simulink model "X31dynamics_03"  (R2014b)
settings: Solver=ode45  StartTime=0.0  StopTime=20  RelTol=1e-3
InitFcn:
  | X31dynamics_03_init
undefined symbols (not defined in the file or in its folder): Newton, Raphson, X31_initC, X31_initR, X31_initX, X31_physical
libraries: QuaternionLib x9, cstblocks x7, simulink x2
settings Model: Creator=EwingKang  LastModifiedBy=5909
settings SolverCC: ZeroCrossAlgorithm=Adaptive
settings DataIOCC: SaveOutput=off  SaveTime=off
settings OptimizationCC: InlineParams=on
settings DebuggingCC: UnderspecifiedInitializationDetection=Classic  MergeDetectMultiDrivingBlocksExec=none  StateNameClashWarn=warning  StrictBusMsg=ErrorOnBusTreatedAsVector
settings ModelReferenceCC: ModelReferenceNumInstancesAllowed=Single  ModelReferencePassRootInputsByReference=off
settings SimscapeCC: EditingMode=Restricted

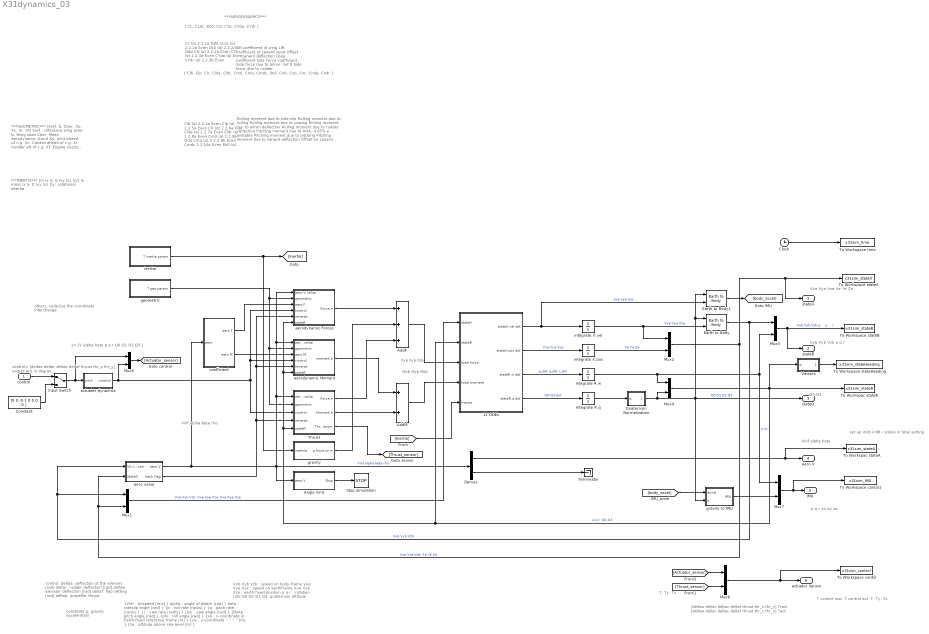
== system X31dynamics_03 ==
  note: Q0-Q3
  note: set up initX initR i sdone in total setting
  note: others:
      | code-lize the coordinate interchange
  note: constants
      | g: gravity acceleration
  note: control:
      |   deltaa: deflection of the ailerons [rad]
      |   deltar: rudder deflection [rad]
      |   deltae: elevator deflection [rad]
      |   deltaf: flap setting [rad]
      |   deltap: propeller thrust
  note: Vxb  Vyb Vzb : speed on body frame
      | Vxe Vye Vze  : speed on earthframe
      | Xxe Xye Xze  : earth fixed position
      | p q r               : rotation rate
      | Q0 Q1 Q2 Q3: quaternion attitude
  note: Vxb Vyb Vzb
      | p     q     r
  note: Vxe Vye Vze
      | Xe   Ye   Ze
  note: {Vinf    : airspeed [m/s]                                                  }
      |  alpha : angle of attack [rad]                                          }
      |  beta   : sideslip angle [rad]                                           }
      | {p    : roll rate [rad/s]                                                      }
      | {q    : pitch rate [rad/s]                                                   }
      | {r     : yaw rate [rad/s]                                                    }
      | {psi    : yaw angle [rad]                                                  }
      | {theta : pitch angle [rad]                                                }
      | {phi    : roll angle [rad]                                                   }
      | {xe   : x-coordinate in Earth-fixed reference frame [m]  }
      | {ye   : y-coordinate ''     ''          ''      ''  [m]                     }
      | {ze   : altitude above sea-level [m]                                }
  note: control= [deltaa deltar deltac deltaf thrust thr_z thr_y]
      | angles are in degree
  note: x= [V alpha beta p q r Q0 Q1 Q2 Q3 ]
  note: Mxb Myb Mzb
  note: Fxb Fyb Fzb
  note: Vinf
      | alpha
      | beta
      | rho
  note: ***AERODYNAMICS***
  note: ***INERTIA***
      | [m Ix Iy Iz Ixy Ixz Iyz]
      | m : mass
      | Ix Iy Iz Ixy Ixz Izy: rotational intertia
  note: ***GEOMETRIC***
      |  [Sref, b, Cbar, Xp, Xc, Xr, Xt]
      |
      | Sref : reference wing area
      | b: Wing span
      | Cbar: Mean aerodynamic chord
      | Xp: pilot ahead of c.g.
      | Xc: Canard ahead of c.g.
      | Xr: Rudder aft of c.g.
      | Xt: Engine nozzle after of c.g.
  note: Rolling moment due to side-slip
      | Rolling moment due to rolling
      | Rolling moment due to yawing
      | Rolling moment due to ailron deflection
      | Rolling moment due to rudder deflection
      |
      | Pitching moment due to AOA, 4.65% e unstable
      | Pitching moment due to pitching
      | Pitching moment due to canard deflection
      | Offset on canard deflection
      |
      | Yawing moment due to side-slip
      | Yawing moment due to rolling
      | Yawing moment due to yawing
      | Yawing moment due to ailron deflection
      | Yawing moment due to rudder deflection
  note: Lift coefficient of wing
      | Lift coefficient of canard input
      | Offset on canard deflection
      | Drag coefficient
      | Side Force coefficient
      | Side force due to ailron, set 0
      | Side force due to rudder
  note: Clb    (α) 2.2.4a Even
      | Clp    (α) 2.2.5a Even
      | Clr     (α) 2.2.6a Odd
      | Clda  (α) 2.2.7a Even
      | Cldr   (α) 2.2.8a Even
      |
      | Cm0  (α) 2.2.9a Odd
      | Cmq  (α) 3 2.2.9b Even
      | Cmdc      2.2.10a Even
      | Dc0   (α) 2.2.2/10b Odd
      |
      | Cnb  (α) 2.2.4b Even
      | Cnp  (α) 2.2.5b Odd
      | Cnr   (α) 2.2.6b Even
      | Cnda(α) 2.2.7b Even
      | Cndr (α) 2.2.8b Even
  note: CL     (α) 2.2.1a Odd
      | CLdc (α)  2.2.2a Even
      | Dc0   (α)  2.2.2/l0b Odd
      | CD     (α)  2.2.1b Even
      | CYb   (α) 2.2.3a Even
      | CYda (α)            Even
      | CYdr  (α) 2.2.3b Even
  note: [ CL, CLdc, Dc0, CD, CYp, CYda, CYdr ]
  note: [ Clb, Clp, Clr, Clda, Cldr, Cm0, Cmq, Cmdc, Dc0, Cnb, Cnp, Cnr, Cnda, Cndr ]
  note: Vinf
      | alpha
      | beta
  note: T, Ty, Tz
  note: [deltaa deltar deltac deltaf thrust thr_z thr_y] 7raw
      | [deltaa deltar deltac deltaf thrust thr_z thr_y] 7act
  note: 7 contorl raw, 7 control act, T, Ty, Tz
  note: p q r ax ay az
  control : Inport  PortDimensions=7
  12 ODEs : Subsystem
  AddF : Sum  Inputs=+++
  AddM : Sum
  Angle limit : Subsystem
  Clock : Clock
  Constant : Constant  Value=[0 0 -0.1 0 0 0 0 ]
  Demux : Demux  Outputs=[3 1 ]
  Earth to Body : QuaternionLib/Earth to Body
  Earth to Body1 : QuaternionLib/Earth to Body
  Input Switch : ManualSwitch
  Integrate R.q : Integrator  InitialCondition=X31_initR.q
  Integrate R.w : Integrator  InitialCondition=X31_initR.w
  Mux{1..7} (7 alike) : Mux  Inputs=2
  Quaternion Normalization : Subsystem
  Stop Simulation : Stop
  Terminator : Terminator
  Thrust : Subsystem
  To Workspac stateA : ToWorkspace  VariableName=x31sim_stateA  SaveFormat=Timeseries  SampleTime=-1
  To Workspac stateR : ToWorkspace  VariableName=x31sim_stateR  SaveFormat=Timeseries  SampleTime=-1
  To Workspace contol : ToWorkspace  VariableName=x31sim_control  SaveFormat=Timeseries  SampleTime=-1
  To Workspace contol1 : ToWorkspace  VariableName=x31sim_IMU  SaveFormat=Timeseries  SampleTime=-1
  To Workspace stateB : ToWorkspace  VariableName=x31sim_stateB  SaveFormat=Timeseries  SampleTime=-1
  To Workspace stateHeading : ToWorkspace  VariableName=x31sim_stateHeading  SaveFormat=Timeseries  SampleTime=-1
  To Workspace stateX : ToWorkspace  VariableName=x31sim_stateX  SaveFormat=Timeseries  SampleTime=-1
  To Workspace time : ToWorkspace  VariableName=x31sim_time  SaveFormat=Timeseries  SampleTime=-1
  Vectors : Subsystem
  actuater dynamics : Subsystem
  aero value : Subsystem
  aerodynamic Forces : Subsystem
  aerodynamic Moment : Subsystem
  coefficient : Subsystem
  geometric : Subsystem
  gravity : Subsystem
  gravity to IMU : Subsystem
  inertia : Subsystem
  integrate X.pos : Integrator  InitialCondition=X31_initX.pos
  integrate X.vel : Integrator  InitialCondition=X31_initX.vel
  stateX : Outport
  stateB : Outport  Port=2
  stateQ : Outport  Port=3
  aero V : Outport  Port=4
  IMU : Outport  Port=5
  actuator Sensor : Outport  Port=6
  wires:
  12 ODEs/1(stateX.vel dot) -> Earth to Body1/2, integrate X.vel/1  "axe aye aze"
  12 ODEs/3("stateR.w dot ") -> Integrate R.w/1  "p_dot q_dot r_dot"
  Mux2/1 -> To Workspace stateX/1, stateX/1, aero value/2(StateX), Mux1/2  "Vxe Vye Vze  Xe Ye Ze"
  Earth to Body/1 -> Mux3/1, aero value/1(Vb vector), Mux1/1  "Vxb Vyb Vzb"
  Mux1/1 -> 12 ODEs/1(stateX)  "Vxb Vyb Vzb  Vxe Vye Vze  Xxe Xye Xze"
  aerodynamic Forces/1(Force e) -> AddF/1
  gravity/1(g force on e) -> AddF/2
  aerodynamic Moment/1(moment b) -> AddM/1
  AddM/1 -> 12 ODEs/4(total moment)
  AddF/1 -> 12 ODEs/3(total force)
  geometric/1(7 geo param) -> Thrust/2(geometric), aerodynamic Moment/2(geometric), aerodynamic Forces/2(geometric)
  coefficient/1(aero F) -> aerodynamic Forces/3(aero F)
  Input Switch/1 -> actuater dynamics/1(cmd), Mux5/1
  aero value/1(aero V) -> coefficient/1(aero), aerodynamic Moment/1(aero V value), aerodynamic Forces/1(aero V value), Thrust/1(aero V value), Angle limit/1(aero V), Demux/1  "Vinf alpha beta rho"
  inertia/1(7 inertia param) -> [Inertia], gravity/1(inertria)
  Clock/1 -> To Workspace time/1
  aero value/2(back flag) -> aerodynamic Moment/5(reverse), aerodynamic Forces/5(reverse), Thrust/4(reverse)
  Mux4/1 -> To Workspac stateR/1, aerodynamic Moment/6(stateR), aerodynamic Forces/6(stateR), Thrust/5(stateR), 12 ODEs/2(stateR), Vectors/1(q)  "p q r  Q0-Q3"
  Quaternion Normalization/1(qnorm) -> Earth to Body1/1, Earth to Body/1, gravity to IMU/2(q), stateQ/1, Mux4/2  "Q0 Q1 Q2 Q3"
  integrate X.vel/1 -> Earth to Body/2, Mux2/1  "Vxe Vye Vze"
  Integrate R.w/1 -> Mux3/2, Mux7/1, Mux4/1  "p q r"
  Integrate R.q/1 -> Quaternion Normalization/1(q)
  actuater dynamics/1(control) -> aerodynamic Moment/4(control), aerodynamic Forces/4(control), Thrust/3(control), Mux5/2
  Mux5/1 -> [Actuator_sensor]
  [Inertia] -> 12 ODEs/5(Inertia)
  Mux3/1 -> To Workspace stateB/1, stateB/1  "Vxb Vyb Vzb p     q     r"
  Constant/1 -> Input Switch/2
  control/1 -> Input Switch/1
  coefficient/2(aero M) -> aerodynamic Moment/3(aero M)
  Thrust/2(Moment b) -> AddM/2
  Thrust/1(Force e) -> AddF/3
  Angle limit/1(Stop) -> Stop Simulation/1
  12 ODEs/2(stateX.pos dot) -> integrate X.pos/1  "Vxe Vye Vze"
  12 ODEs/4(stateR.q dot) -> Integrate R.q/1  "Q0-Q3 dot"
  integrate X.pos/1 -> Mux2/2  "Xe Ye Ze"
  Vectors/1(Vector) -> To Workspace stateHeading/1
  Demux/1 -> To Workspac stateA/1, aero V/1
  Demux/2 -> Terminator/1
  [Thrust_sensor] -> Mux6/2
  Thrust/3(Thrust sensor) -> [Thrust_sensor]
  [Actuator_sensor] -> Mux6/1
  Mux6/1 -> actuator Sensor/1, To Workspace contol/1
  Mux7/1 -> IMU/1, To Workspace contol1/1
  Earth to Body1/1 -> [body_accel]
  [body_accel] -> gravity to IMU/1(accel)
  gravity to IMU/1(IMU) -> Mux7/2

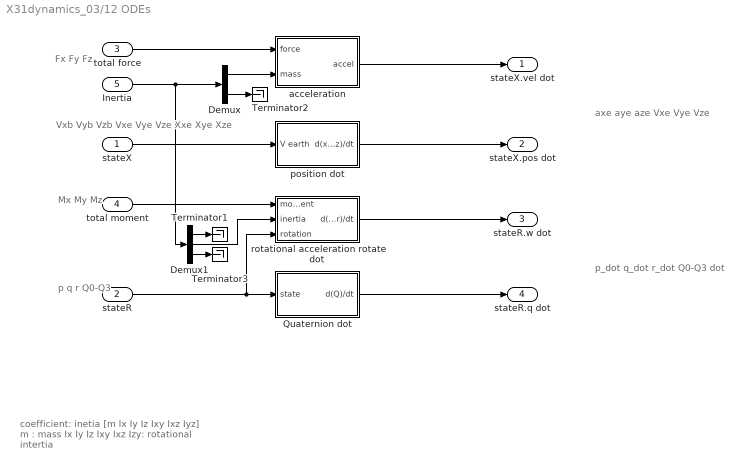
== system X31dynamics_03/12 ODEs ==
  note: p_dot q_dot r_dot
      | Q0-Q3 dot
  note: axe aye aze
      | Vxe Vye Vze
  note: Vxb Vyb Vzb Vxe Vye Vze Xxe Xye Xze
  note: Mx My Mz
  note: Fx Fy Fz
  note: p q r Q0-Q3
  note: coefficient: inetia
      | [m Ix Iy Iz Ixy Ixz Iyz]
      | m : mass
      | Ix Iy Iz Ixy Ixz Izy: rotational intertia
  stateX : Inport
  stateR : Inport  Port=2
  total force : Inport  Port=3
  total moment : Inport  Port=4
  Inertia : Inport  Port=5
  Demux : Demux  Outputs=[1 6]
  Demux1 : Demux  Outputs=[1 3 3]
  Quaternion dot : Subsystem
  Terminator1 : Terminator
  Terminator2 : Terminator
  Terminator3 : Terminator
  acceleration : Subsystem
  position dot : Subsystem
  rotational acceleration rotate dot : Subsystem
  stateX.vel dot : Outport
  stateX.pos dot : Outport  Port=2
  "stateR.w dot " : Outport  Port=3
  stateR.q dot : Outport  Port=4
  wires:
  Inertia/1 -> Demux1/1, Demux/1
  total moment/1 -> rotational acceleration rotate dot/1(moment)
  total force/1 -> acceleration/1(force)
  stateR/1 -> rotational acceleration rotate dot/3(rotation), Quaternion dot/1(state)
  acceleration/1(accel) -> stateX.vel dot/1
  position dot/1(d(xyz)/dt) -> stateX.pos dot/1
  rotational acceleration rotate dot/1(d(pqr)/dt) -> "stateR.w dot "/1
  stateX/1 -> position dot/1(V earth)
  Demux/1 -> acceleration/2(mass)
  Demux/2 -> Terminator2/1
  Demux1/2 -> rotational acceleration rotate dot/2(inertia)
  Demux1/1 -> Terminator1/1
  Demux1/3 -> Terminator3/1
  Quaternion dot/1(d(Q)/dt) -> stateR.q dot/1

== system X31dynamics_03/Angle limit ==
  note: Vinf
      | alpha
      | beta
      | rho
  aero V : Inport
  85 degree : simulink/Logic and Bit Operations/Compare To Constant  relop=>  const=85 * pi / 180  OutDataTypeStr=boolean
  85 degree1 : simulink/Logic and Bit Operations/Compare To Constant  relop=>  const=80 * pi / 180  OutDataTypeStr=boolean
  Abs : Abs
  Abs1 : Abs
  Any violation : Logic  Operator=OR  AllPortsSameDT=off  OutDataTypeStr=boolean
  Assertion : Assertion  AssertionFailFcn=warning('large angle in x31dynamics_03')  StopWhenAssertionFail=off
  Logical Operator : Logic  Operator=NOT  AllPortsSameDT=off  OutDataTypeStr=boolean
  alpha : Fcn  Expr=u(2)
  beta : Fcn  Expr=u(3)
  Stop : Outport
  wires:
  aero V/1 -> alpha/1, beta/1
  85 degree/1 -> Any violation/1
  alpha/1 -> Abs/1
  beta/1 -> Abs1/1
  85 degree1/1 -> Any violation/2
  Abs/1 -> 85 degree/1
  Abs1/1 -> 85 degree1/1
  Any violation/1 -> Logical Operator/1, Stop/1
  Logical Operator/1 -> Assertion/1

== system X31dynamics_03/Quaternion Normalization ==
  q : Inport  PortDimensions=4
  Product : Product  Inputs=*/  SaturateOnIntegerOverflow=on  RndMeth=Zero  InputSameDT=on  OutDataTypeStr=Inherit: Same as first input
  Square : Math  Operator=square  SaturateOnIntegerOverflow=on
  Square Root : Sqrt  Operator=signedSqrt  AlgorithmType=Newton-Raphson  SaturateOnIntegerOverflow=on
  Sum : Sum  Inputs=1  SaturateOnIntegerOverflow=on  InputSameDT=on  OutDataTypeStr=Inherit: Same as first input
  qnorm : Outport
  wires:
  Product/1 -> qnorm/1
  Square Root/1 -> Product/2
  Square/1 -> Sum/1
  Sum/1 -> Square Root/1
  q/1 -> Product/1, Square/1

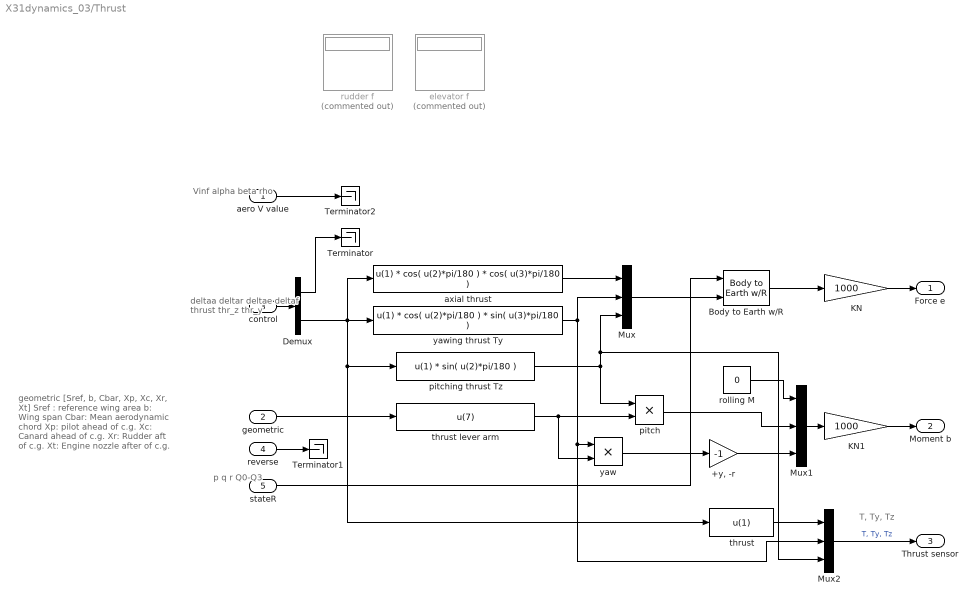
== system X31dynamics_03/Thrust ==
  note: T, Ty, Tz
  note: Vinf alpha beta rho
  note: p q r
      | Q0-Q3
  note: geometric
      |  [Sref, b, Cbar, Xp, Xc, Xr, Xt]
      |
      | Sref : reference wing area
      | b: Wing span
      | Cbar: Mean aerodynamic chord
      | Xp: pilot ahead of c.g.
      | Xc: Canard ahead of c.g.
      | Xr: Rudder aft of c.g.
      | Xt: Engine nozzle after of c.g.
  note: deltaa deltar deltae deltaf
      | thrust thr_z thr_y
  aero V value : Inport
  geometric : Inport  Port=2
  control : Inport  Port=3
  reverse : Inport  Port=4
  stateR : Inport  Port=5
  " thrust" : Fcn  Expr=u(1)
  "+y, -r" : Gain  Gain=-1
  Body to Earth w/R : QuaternionLib/Body to Earth w//R
  Demux : Demux  Outputs=[4 3]
  KN : Gain  Gain=1000
  KN1 : Gain  Gain=1000
  Mux : Mux  Inputs=3
  Mux1 : Mux  Inputs=3
  Mux2 : Mux  Inputs=3
  Terminator : Terminator
  Terminator1 : Terminator
  Terminator2 : Terminator
  axial thrust : Fcn  Expr="u(1) * cos( u(2)*pi/180  ) * cos( u(3)*pi/180  )"
  elevator f : Display  Commented=on
  pitch : Product
  pitching thrust Tz : Fcn  Expr=u(1) * sin( u(2)*pi/180 )
  rolling M : Constant  Value=0
  rudder f : Display  Commented=on
  thrust lever arm : Fcn  Expr=u(7)
  yaw : Product
  yawing thrust Ty : Fcn  Expr=u(1) * cos( u(2)*pi/180 ) * sin( u(3)*pi/180 )
  Force e : Outport
  Moment b : Outport  Port=2
  Thrust sensor : Outport  Port=3
  wires:
  control/1 -> Demux/1
  Body to Earth w/R/1 -> KN/1
  Demux/1 -> Terminator/1
  yawing thrust Ty/1 -> Mux/2, Mux2/2, yaw/1
  axial thrust/1 -> Mux/1
  pitching thrust Tz/1 -> Mux2/3, Mux/3, pitch/1
  Mux/1 -> Body to Earth w/R/2
  stateR/1 -> Body to Earth w/R/1
  Demux/2 -> " thrust"/1, pitching thrust Tz/1, axial thrust/1, yawing thrust Ty/1
  reverse/1 -> Terminator1/1
  aero V value/1 -> Terminator2/1
  geometric/1 -> thrust lever arm/1
  thrust lever arm/1 -> yaw/2, pitch/2
  yaw/1 -> "+y, -r"/1
  pitch/1 -> Mux1/2
  rolling M/1 -> Mux1/1
  Mux1/1 -> KN1/1
  KN/1 -> Force e/1
  KN1/1 -> Moment b/1
  "+y, -r"/1 -> Mux1/3
  Mux2/1 -> Thrust sensor/1  "T, Ty, Tz"
  " thrust"/1 -> Mux2/1

== system X31dynamics_03/Vectors ==
  q : Inport
  1,0,0 : Subsystem
  1,0,1 : Subsystem
  Body to Earth w/R1 : QuaternionLib/Body to Earth w//R
  Body to Earth w/R2 : QuaternionLib/Body to Earth w//R
  Mux6 : Mux  Inputs=2
  Vector : Outport
  wires:
  1,0,0/1(1,0,0) -> Body to Earth w/R1/2
  Body to Earth w/R1/1 -> Mux6/1
  q/1 -> Body to Earth w/R1/1, Body to Earth w/R2/1  "p q r  Q0-Q3"
  Mux6/1 -> Vector/1
  Body to Earth w/R2/1 -> Mux6/2
  1,0,1/1(0,1,0) -> Body to Earth w/R2/2

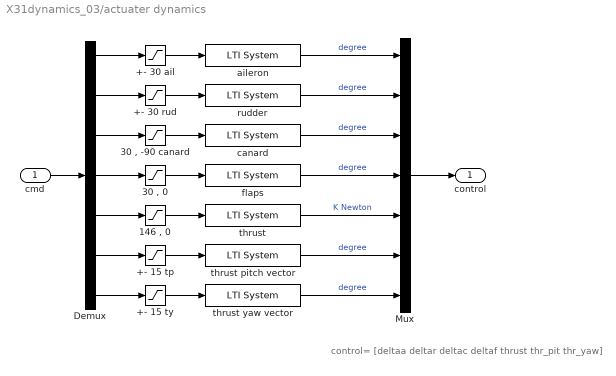
== system X31dynamics_03/actuater dynamics ==
  note: control= [deltaa deltar deltac deltaf thrust thr_pit thr_yaw]
  cmd : Inport
  +- 15 tp : Saturate  UpperLimit=15  LowerLimit=-15
  +- 15 ty : Saturate  UpperLimit=15  LowerLimit=-15
  +- 30 ail : Saturate  UpperLimit=30  LowerLimit=-30
  +- 30 rud : Saturate  UpperLimit=30  LowerLimit=-30
  "146 , 0" : Saturate  UpperLimit=146  LowerLimit=0
  "30 , -90 canard" : Saturate  UpperLimit=30  LowerLimit=-90
  "30 , 0" : Saturate  UpperLimit=30  LowerLimit=0
  Demux : Demux  Outputs=7
  Mux : Mux  Inputs=7
  aileron : cstblocks/LTI System  sys=tf(30,[1 30])  IC=[]
  canard : cstblocks/LTI System  sys=tf(30,[1 30])  IC=[]
  flaps : cstblocks/LTI System  sys=tf(30,[1 30])  IC=[]
  rudder : cstblocks/LTI System  sys=tf(30,[1 30])  IC=[]
  thrust : cstblocks/LTI System  sys=ss(-1/3, 1, 1/3, 0)  IC=[X31_initC.thrust*3]
  thrust pitch vector : cstblocks/LTI System  sys=tf(30,[1 30])  IC=[]
  thrust yaw vector : cstblocks/LTI System  sys=tf(30,[1 30])  IC=[]
  control : Outport
  wires:
  cmd/1 -> Demux/1
  Demux/4 -> "30 , 0"/1
  Demux/3 -> "30 , -90 canard"/1
  Demux/2 -> +- 30 rud/1
  Demux/1 -> +- 30 ail/1
  Demux/5 -> "146 , 0"/1
  Demux/6 -> +- 15 tp/1
  Demux/7 -> +- 15 ty/1
  thrust yaw vector/1 -> Mux/7  "degree"
  thrust pitch vector/1 -> Mux/6  "degree"
  thrust/1 -> Mux/5  "K Newton"
  flaps/1 -> Mux/4  "degree"
  canard/1 -> Mux/3  "degree"
  rudder/1 -> Mux/2  "degree"
  aileron/1 -> Mux/1  "degree"
  Mux/1 -> control/1
  +- 30 ail/1 -> aileron/1
  +- 30 rud/1 -> rudder/1
  "30 , -90 canard"/1 -> canard/1
  "30 , 0"/1 -> flaps/1
  "146 , 0"/1 -> thrust/1
  +- 15 tp/1 -> thrust pitch vector/1
  +- 15 ty/1 -> thrust yaw vector/1

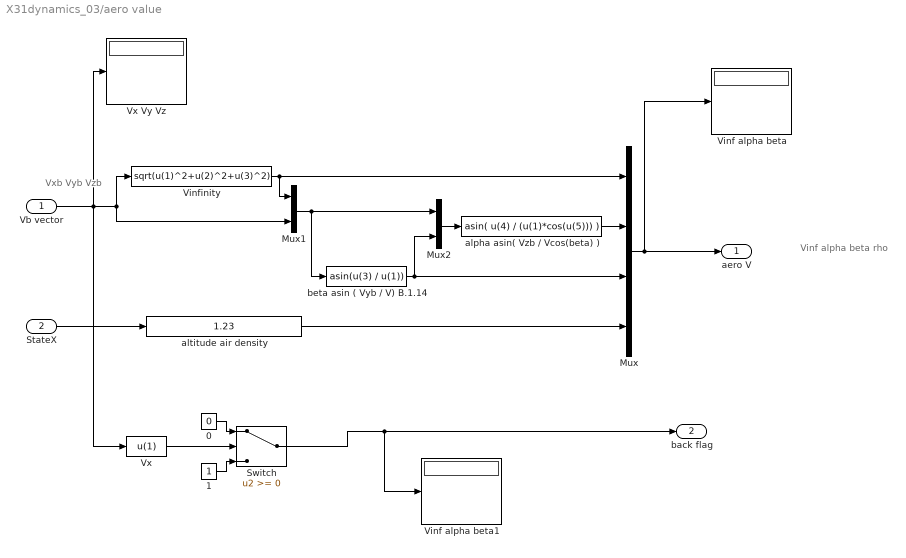
== system X31dynamics_03/aero value ==
  note: Vinf
      | alpha
      | beta
      | rho
  note: Vxb Vyb Vzb
  Vb vector : Inport
  StateX : Inport  Port=2
  0 : Constant  Value=0
  1 : Constant
  Mux : Mux
  Mux1 : Mux  Inputs=2
  Mux2 : Mux  Inputs=2
  Switch : Switch  ZeroCross=off
  Vinf alpha beta : Display
  Vinf alpha beta1 : Display
  Vinfinity : Fcn  Expr=sqrt(u(1)^2+u(2)^2+u(3)^2)
  Vx : Fcn  Expr=u(1)
  Vx Vy Vz : Display
  alpha asin( Vzb / Vcos(beta) ) : Fcn  Expr=asin( u(4) / (u(1)*cos(u(5))) )
  altitude air density : Fcn  Expr=1.23
  beta asin ( Vyb / V) B.1.14 : Fcn  Expr=asin(u(3) / u(1))
  aero V : Outport
  back flag : Outport  Port=2
  wires:
  Vb vector/1 -> Vx/1, Vx Vy Vz/1, Vinfinity/1, Mux1/2
  Vinfinity/1 -> Mux1/1, Mux/1
  beta asin ( Vyb / V) B.1.14/1 -> Mux/3, Mux2/2
  Mux/1 -> aero V/1, Vinf alpha beta/1
  alpha asin( Vzb / Vcos(beta) )/1 -> Mux/2
  Vx/1 -> Switch/2
  0/1 -> Switch/1
  1/1 -> Switch/3
  Switch/1 -> Vinf alpha beta1/1, back flag/1
  Mux1/1 -> beta asin ( Vyb / V) B.1.14/1, Mux2/1
  altitude air density/1 -> Mux/4
  StateX/1 -> altitude air density/1
  Mux2/1 -> alpha asin( Vzb / Vcos(beta) )/1

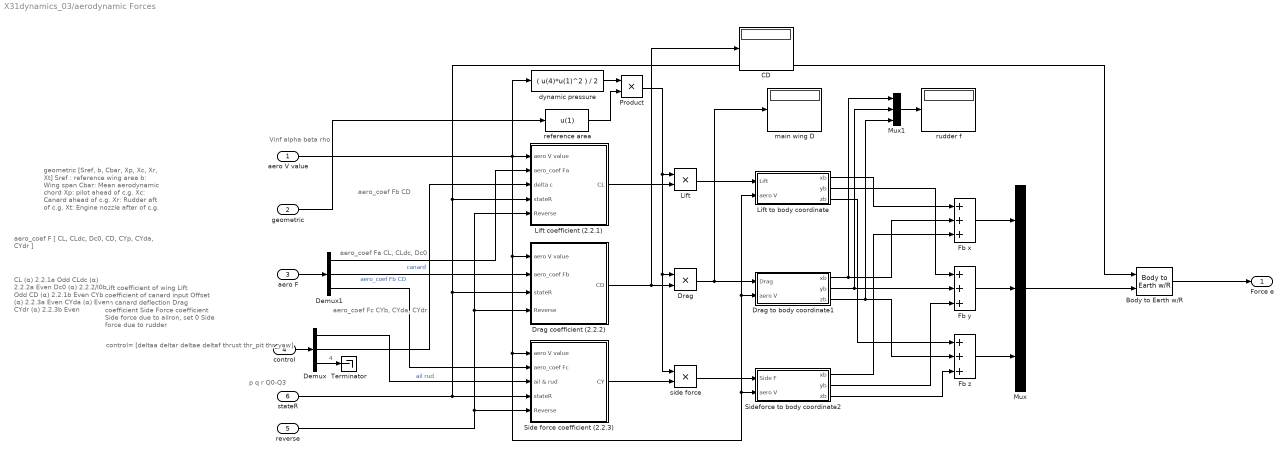
== system X31dynamics_03/aerodynamic Forces ==
  note: Vinf alpha beta rho
  note: p q r
      | Q0-Q3
  note: Lift coefficient of wing
      | Lift coefficient of canard input
      | Offset on canard deflection
      | Drag coefficient
      | Side Force coefficient
      | Side force due to ailron, set 0
      | Side force due to rudder
  note: CL     (α) 2.2.1a Odd
      | CLdc (α)  2.2.2a Even
      | Dc0   (α)  2.2.2/l0b Odd
      | CD     (α)  2.2.1b Even
      | CYb   (α) 2.2.3a Even
      | CYda (α)            Even
      | CYdr  (α) 2.2.3b Even
  note: aero_coef F
      | [ CL, CLdc, Dc0, CD, CYp, CYda, CYdr ]
  note: geometric
      |  [Sref, b, Cbar, Xp, Xc, Xr, Xt]
      |
      | Sref : reference wing area
      | b: Wing span
      | Cbar: Mean aerodynamic chord
      | Xp: pilot ahead of c.g.
      | Xc: Canard ahead of c.g.
      | Xr: Rudder aft of c.g.
      | Xt: Engine nozzle after of c.g.
  note: aero_coef Fa
      | CL, CLdc, Dc0
  note: aero_coef Fc
      | CYb, CYda, CYdr
  note: aero_coef Fb
      | CD
  note: control= [deltaa deltar deltae deltaf thrust thr_pit thr_yaw]
  aero V value : Inport
  geometric : Inport  Port=2
  aero F : Inport  Port=3
  control : Inport  Port=4
  reverse : Inport  Port=5
  stateR : Inport  Port=6
  Body to Earth w/R : QuaternionLib/Body to Earth w//R
  CD : Display
  Demux : Demux  Outputs=[2 1 4]
  Demux1 : Demux  Outputs=[3 1 3]
  Drag : Product
  Drag coefficient (2.2.2) : Subsystem
  Drag to body coordinate1 : Subsystem
  Fb x : Sum  Inputs=+++
  Fb y : Sum  Inputs=+++
  Fb z : Sum  Inputs=+++
  Lift : Product
  Lift coefficient (2.2.1) : Subsystem
  Lift to body coordinate : Subsystem
  Mux : Mux  Inputs=3
  Mux1 : Mux  Inputs=3
  Product : Product
  Side force coefficient (2.2.3) : Subsystem
  Sideforce to body coordinate2 : Subsystem
  Terminator : Terminator
  dynamic pressure : Fcn  Expr=( u(4)*u(1)^2 ) / 2
  main wing D : Display
  reference area : Fcn  Expr=u(1)
  rudder f : Display
  side force : Product
  Force e : Outport
  wires:
  control/1 -> Demux/1
  Demux/2 -> Lift coefficient (2.2.1)/3(delta c)  "canard"
  Body to Earth w/R/1 -> Force e/1
  Demux/3 -> Terminator/1  "4"
  stateR/1 -> Body to Earth w/R/1, Lift coefficient (2.2.1)/4(stateR), Drag coefficient (2.2.2)/3(stateR), Side force coefficient (2.2.3)/4(stateR)
  reverse/1 -> Lift coefficient (2.2.1)/5(Reverse), Drag coefficient (2.2.2)/4(Reverse), Side force coefficient (2.2.3)/5(Reverse)
  aero V value/1 -> Lift to body coordinate/2(aero V), Drag to body coordinate1/2(aero V), Sideforce to body coordinate2/2(aero V), Side force coefficient (2.2.3)/1(aero V value), Drag coefficient (2.2.2)/1(aero V value), dynamic pressure/1, Lift coefficient (2.2.1)/1(aero V value)
  Demux1/1 -> Lift coefficient (2.2.1)/2(aero_coef Fa)
  Demux/1 -> Side force coefficient (2.2.3)/3(ail & rud)  "ail rud"
  aero F/1 -> Demux1/1
  Demux1/3 -> Side force coefficient (2.2.3)/2(aero_coef Fc)
  Demux1/2 -> Drag coefficient (2.2.2)/2(aero_coef Fb)  "aero_coef Fb CD"
  geometric/1 -> reference area/1
  dynamic pressure/1 -> Product/1
  reference area/1 -> Product/2
  Product/1 -> side force/1, Drag/1, Lift/1
  Lift coefficient (2.2.1)/1(CL) -> Lift/2
  Drag coefficient (2.2.2)/1(CD) -> CD/1, Drag/2
  Side force coefficient (2.2.3)/1(CY) -> side force/2
  Lift/1 -> Lift to body coordinate/1(Lift)
  side force/1 -> Sideforce to body coordinate2/1(Side F)
  Drag/1 -> main wing D/1, Drag to body coordinate1/1(Drag)
  Lift to body coordinate/1(xb) -> Fb x/1
  Drag to body coordinate1/1(xb) -> Mux1/1, Fb x/2
  Sideforce to body coordinate2/1(xb) -> Fb x/3
  Lift to body coordinate/2(yb) -> Fb y/1
  Lift to body coordinate/3(zb) -> Fb z/1
  Drag to body coordinate1/3(zb) -> Fb z/2, Mux1/3
  Sideforce to body coordinate2/2(yb) -> Fb y/3
  Drag to body coordinate1/2(yb) -> Mux1/2, Fb y/2
  Sideforce to body coordinate2/3(zb) -> Fb z/3
  Fb z/1 -> Mux/3
  Fb x/1 -> Mux/1
  Fb y/1 -> Mux/2
  Mux/1 -> Body to Earth w/R/2
  Mux1/1 -> rudder f/1

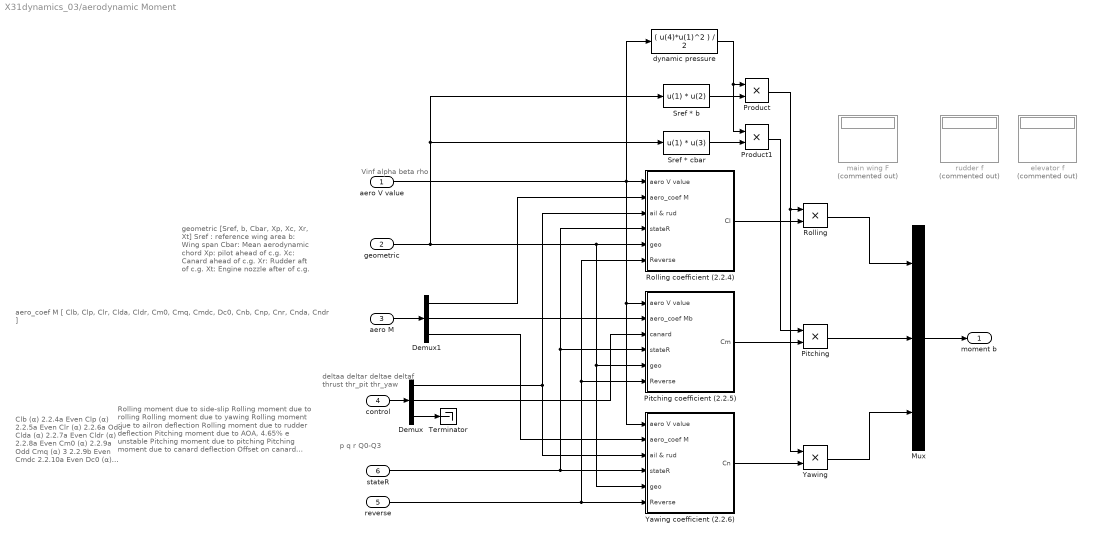
== system X31dynamics_03/aerodynamic Moment ==
  note: Vinf alpha beta rho
  note: p q r
      | Q0-Q3
  note: geometric
      |  [Sref, b, Cbar, Xp, Xc, Xr, Xt]
      |
      | Sref : reference wing area
      | b: Wing span
      | Cbar: Mean aerodynamic chord
      | Xp: pilot ahead of c.g.
      | Xc: Canard ahead of c.g.
      | Xr: Rudder aft of c.g.
      | Xt: Engine nozzle after of c.g.
  note: Rolling moment due to side-slip
      | Rolling moment due to rolling
      | Rolling moment due to yawing
      | Rolling moment due to ailron deflection
      | Rolling moment due to rudder deflection
      |
      | Pitching moment due to AOA, 4.65% e unstable
      | Pitching moment due to pitching
      | Pitching moment due to canard deflection
      | Offset on canard deflection
      |
      | Yawing moment due to side-slip
      | Yawing moment due to rolling
      | Yawing moment due to yawing
      | Yawing moment due to ailron deflection
      | Yawing moment due to rudder deflection
  note: Clb    (α) 2.2.4a Even
      | Clp    (α) 2.2.5a Even
      | Clr     (α) 2.2.6a Odd
      | Clda  (α) 2.2.7a Even
      | Cldr   (α) 2.2.8a Even
      |
      | Cm0  (α) 2.2.9a Odd
      | Cmq  (α) 3 2.2.9b Even
      | Cmdc      2.2.10a Even
      | Dc0   (α) 2.2.2/10b Odd
      |
      | Cnb  (α) 2.2.4b Even
      | Cnp  (α) 2.2.5b Odd
      | Cnr   (α) 2.2.6b Even
      | Cnda(α) 2.2.7b Even
      | Cndr (α) 2.2.8b Even
  note: aero_coef M
      | [ Clb, Clp, Clr, Clda, Cldr, Cm0, Cmq, Cmdc, Dc0, Cnb, Cnp, Cnr, Cnda, Cndr ]
  note: deltaa
      | deltar
      | deltae
      | deltaf
      | thrust
      | thr_pit
      | thr_yaw
  aero V value : Inport
  geometric : Inport  Port=2
  aero M : Inport  Port=3
  control : Inport  Port=4
  reverse : Inport  Port=5
  stateR : Inport  Port=6
  Demux : Demux  Outputs=[2 1 4]
  Demux1 : Demux  Outputs=[5 4 5]
  Mux : Mux  Inputs=3
  Pitching : Product
  Pitching coefficient (2.2.5) : Subsystem
  Product : Product
  Product1 : Product
  Rolling : Product
  Rolling coefficient (2.2.4) : Subsystem
  Sref * b : Fcn  Expr=u(1) * u(2)
  Sref * cbar : Fcn  Expr=u(1) * u(3)
  Terminator : Terminator
  Yawing : Product
  Yawing coefficient (2.2.6) : Subsystem
  dynamic pressure : Fcn  Expr=( u(4)*u(1)^2 ) / 2
  elevator f : Display  Commented=on
  main wing F : Display  Commented=on
  rudder f : Display  Commented=on
  moment b : Outport
  wires:
  control/1 -> Demux/1
  Mux/1 -> moment b/1
  Demux/3 -> Terminator/1
  stateR/1 -> Rolling coefficient (2.2.4)/4(stateR), Pitching coefficient (2.2.5)/4(stateR), Yawing coefficient (2.2.6)/4(stateR)
  reverse/1 -> Yawing coefficient (2.2.6)/6(Reverse), Pitching coefficient (2.2.5)/6(Reverse), Rolling coefficient (2.2.4)/6(Reverse)
  aero V value/1 -> dynamic pressure/1, Rolling coefficient (2.2.4)/1(aero V value), Pitching coefficient (2.2.5)/1(aero V value), Yawing coefficient (2.2.6)/1(aero V value)
  Demux1/1 -> Rolling coefficient (2.2.4)/2(aero_coef M)
  aero M/1 -> Demux1/1
  Demux1/3 -> Yawing coefficient (2.2.6)/2(aero_coef M)
  Demux1/2 -> Pitching coefficient (2.2.5)/2(aero_coef Mb)
  geometric/1 -> Sref * b/1, Sref * cbar/1, Rolling coefficient (2.2.4)/5(geo), Pitching coefficient (2.2.5)/5(geo), Yawing coefficient (2.2.6)/5(geo)
  dynamic pressure/1 -> Product1/1, Product/1
  Sref * b/1 -> Product/2
  Product/1 -> Yawing/1, Rolling/1
  Rolling coefficient (2.2.4)/1(Cl) -> Rolling/2
  Pitching coefficient (2.2.5)/1(Cm) -> Pitching/2
  Yawing coefficient (2.2.6)/1(Cn) -> Yawing/2
  Yawing/1 -> Mux/3
  Rolling/1 -> Mux/1
  Pitching/1 -> Mux/2
  Demux/1 -> Yawing coefficient (2.2.6)/3(ail & rud), Rolling coefficient (2.2.4)/3(ail & rud)
  Demux/2 -> Pitching coefficient (2.2.5)/3(canard)
  Sref * cbar/1 -> Product1/2
  Product1/1 -> Pitching/1

== system X31dynamics_03/coefficient ==
  note: Rolling moment due to side-slip
      | Rolling moment due to rolling
      | Rolling moment due to yawing
      | Rolling moment due to ailron deflection
      | Rolling moment due to rudder deflection
      |
      | Pitching moment due to AOA, 4.65% e unstable
      | Pitching moment due to pitching
      | Pitching moment due to canard deflection
      | Offset on canard deflection
      |
      | Yawing moment due to side-slip
      | Yawing moment due to rolling
      | Yawing moment due to yawing
      | Yawing moment due to ailron deflection
      | Yawing moment due to rudder deflection
  note: Lift coefficient of wing
      | Lift coefficient of canard input
      | Offset on canard deflection
      | Drag coefficient
      | Side Force coefficient
      | Side force due to ailron, set 0
      | Side force due to rudder
  note: Clb    (α) 2.2.4a Even
      | Clp    (α) 2.2.5a Even
      | Clr     (α) 2.2.6a Odd
      | Clda  (α) 2.2.7a Even
      | Cldr   (α) 2.2.8a Even
      |
      | Cm0  (α) 2.2.9a Odd
      | Cmq  (α) 3 2.2.9b Even
      | Cmdc      2.2.10a Even
      | Dc0   (α) 2.2.2/10b Odd
      |
      | Cnb  (α) 2.2.4b Even
      | Cnp  (α) 2.2.5b Odd
      | Cnr   (α) 2.2.6b Even
      | Cnda(α) 2.2.7b Even
      | Cndr (α) 2.2.8b Even
  note: CL     (α) 2.2.1a Odd
      | CLdc (α)  2.2.2a Even
      | Dc0   (α)  2.2.2/l0b Odd
      | CD     (α)  2.2.1b Even
      | CYb   (α) 2.2.3a Even
      | CYda (α)            Even
      | CYdr  (α) 2.2.3b Even
  note: beta
  note: alpha
  note: [ CL, CLdc, Dc0, CD, CYp, CYda, CYdr ]
  note: [ Clb, Clp, Clr, Clda, Cldr, Cm0, Cmq, Cmdc, Dc0, Cnb, Cnp, Cnr, Cnda, Cndr ]
  aero : Inport
  CYda : Constant  Value=0
  Demux : Demux
  Demux1 : Demux  Outputs=10
  Demux2 : Demux  Outputs=10
  Mux1 : Mux  Inputs=14
  Mux6 : Mux  Inputs=7
  Vinf : Terminator
  aero F disp : Display
  aero M disp : Display
  aerodynamic coefficient : MATLAB Function  TreatAsAtomicUnit=on
  alpha : Display
  beta : Terminator
  rho : Terminator
  aero F : Outport
  aero M : Outport  Port=2
  wires:
  Mux6/1 -> aero F disp/1, aero F/1
  aero/1 -> Demux/1
  Demux/1 -> Vinf/1
  Mux1/1 -> aero M disp/1, aero M/1
  aerodynamic coefficient/1(fa) -> Demux1/1
  aerodynamic coefficient/2(fb) -> Demux2/1
  Demux1/1 -> Mux6/1
  Demux1/2 -> Mux6/2
  Demux2/2 -> Mux6/3
  Demux2/1 -> Mux6/4
  Demux1/3 -> Mux6/5
  Demux2/3 -> Mux6/7
  Demux1/4 -> Mux1/1
  Demux1/5 -> Mux1/2
  Demux1/6 -> Mux1/3
  Demux1/7 -> Mux1/4
  Demux1/8 -> Mux1/5
  Demux1/9 -> Mux1/6
  Demux1/10 -> Mux1/8
  Demux2/4 -> Mux1/10
  Demux2/5 -> Mux1/11
  Demux2/6 -> Mux1/12
  Demux2/7 -> Mux1/13
  Demux2/8 -> Mux1/14
  Demux2/10 -> Mux1/9
  Demux2/9 -> Mux1/7
  Demux/3 -> beta/1
  Demux/2 -> alpha/1, aerodynamic coefficient/1(a)
  Demux/4 -> rho/1
  CYda/1 -> Mux6/6

== system X31dynamics_03/geometric ==
  note: geometric
      |  [Sref, b, Cbar, Xp, Xc, Xr, Xt]
      |
      | Sref : reference wing area
      | b: Wing span
      | Cbar: Mean aerodynamic chord
      | Xp: pilot ahead of c.g.
      | Xc: Canard ahead of c.g.
      | Xr: Rudder aft of c.g.
      | Xt: Engine nozzle after of c.g.
  Cbar : Constant  Value=X31_physical.geometry.Cbar
  Mux6 : Mux  Inputs=7
  Sref : Constant  Value=X31_physical.geometry.Sref
  Xc : Constant  Value=X31_physical.geometry.Xc
  Xp : Constant  Value=X31_physical.geometry.Xp
  Xr : Constant  Value=X31_physical.geometry.Xr
  Xt : Constant  Value=X31_physical.geometry.Xt
  b : Constant  Value=X31_physical.geometry.b
  7 geo param : Outport
  wires:
  Mux6/1 -> 7 geo param/1
  Sref/1 -> Mux6/1
  b/1 -> Mux6/2
  Cbar/1 -> Mux6/3
  Xp/1 -> Mux6/4
  Xc/1 -> Mux6/5
  Xr/1 -> Mux6/6
  Xt/1 -> Mux6/7

== system X31dynamics_03/gravity ==
  inertria : Inport
  " mass" : Fcn  Expr=u(1)
  Attitude Switch : ManualSwitch
  Constant : Constant  Value=0
  Gain 7 : Gain  Gain=-1  SaturateOnIntegerOverflow=on  OutDataTypeStr=Inherit: Same as input  ParamDataTypeStr=Inherit: Same as input
  Mux : Mux  Inputs=3
  Mux1 : Mux  Inputs=3
  f=ma : Product  Inputs=**
  grav : Display
  gravity : Constant  Value=9.81
  g force on e : Outport
  wires:
  Attitude Switch/1 -> g force on e/1, grav/1
  gravity/1 -> f=ma/2
  " mass"/1 -> f=ma/1
  Constant/1 -> Mux/1, Mux1/3, Mux1/2, Mux/2
  inertria/1 -> " mass"/1
  f=ma/1 -> Gain 7/1, Mux/3
  Mux/1 -> Attitude Switch/1
  Mux1/1 -> Attitude Switch/2
  Gain 7/1 -> Mux1/1

== system X31dynamics_03/gravity to IMU ==
  accel : Inport
  q : Inport  Port=2
  Add : Sum
  Constant : Constant  Value=0
  Earth to Body : QuaternionLib/Earth to Body
  Mux : Mux  Inputs=3
  gravity accel : Constant  Value=-9.81
  IMU : Outport
  wires:
  Constant/1 -> Mux/1, Mux/2
  gravity accel/1 -> Mux/3
  Mux/1 -> Earth to Body/2
  q/1 -> Earth to Body/1
  accel/1 -> Add/1
  Add/1 -> IMU/1
  Earth to Body/1 -> Add/2

== system X31dynamics_03/inertia ==
  note: inetia
      | [m Ix Iy Iz Ixy Ixz Iyz]
      | m : mass
      | Ix Iy Iz Ixy Ixz Izy: rotational intertia
  Ix : Constant  Value=X31_physical.inertia.Ixx
  Ixy : Constant  Value=X31_physical.inertia.Ixy
  Ixz : Constant  Value=X31_physical.inertia.Ixz
  Iy : Constant  Value=X31_physical.inertia.Iyy
  Iyz : Constant  Value=X31_physical.inertia.Iyz
  Iz : Constant  Value=X31_physical.inertia.Izz
  Mux : Mux  Inputs=2
  Mux1 : Mux  Inputs=2
  Mux2 : Mux  Inputs=2
  Mux6 : Mux
  m : Constant  Value=X31_physical.inertia.mass
  7 inertia param : Outport
  wires:
  Ix/1 -> Mux/1
  Iy/1 -> Mux/2
  Ixz/1 -> Mux2/1
  Iyz/1 -> Mux2/2
  Iz/1 -> Mux1/1
  Ixy/1 -> Mux1/2
  Mux6/1 -> 7 inertia param/1
  m/1 -> Mux6/1
  Mux/1 -> Mux6/2
  Mux1/1 -> Mux6/3
  Mux2/1 -> Mux6/4

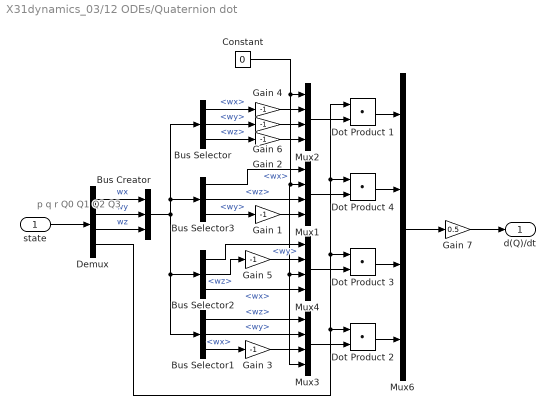
== system X31dynamics_03/12 ODEs/Quaternion dot ==
  note: p q r Q0 Q1 Q2 Q3
  state : Inport
  Bus Creator : BusCreator  Inputs=3
  Bus Selector : BusSelector  OutputSignals=wx,wy,wz
  Bus Selector1 : BusSelector  OutputSignals=wz,wy,wx
  Bus Selector2 : BusSelector  OutputSignals=wy,wz,wx
  Bus Selector3 : BusSelector  OutputSignals=wx,wz,wy
  Constant : Constant  Value=0
  Demux : Demux  Outputs=[1 1 1 4]
  Dot Product {1..4} (4 alike) : DotProduct  InputSameDT=on  OutDataTypeStr=Inherit: Inherit via internal rule
  Gain {1..6} (6 alike) : Gain  Gain=-1  SaturateOnIntegerOverflow=on  OutDataTypeStr=Inherit: Same as input  ParamDataTypeStr=Inherit: Same as input
  Gain 7 : Gain  Gain=0.5  SaturateOnIntegerOverflow=on  OutDataTypeStr=Inherit: Same as input  ParamDataTypeStr=Inherit: Same as input
  Mux{1..4,6} (5 alike) : Mux
  d(Q)/dt : Outport
  wires:
  Mux6/1 -> Gain 7/1
  state/1 -> Demux/1
  Gain 2/1 -> Mux2/4
  Bus Selector/1 -> Gain 4/1  "<wx>"
  Mux2/1 -> Dot Product 1/2
  Mux3/1 -> Dot Product 2/2
  Mux4/1 -> Dot Product 3/2
  Demux/1 -> Bus Creator/1  "wx"
  Demux/2 -> Bus Creator/2  "wy"
  Demux/3 -> Bus Creator/3  "wz"
  Gain 5/1 -> Mux4/2
  Gain 3/1 -> Mux3/3
  Mux1/1 -> Dot Product 4/2
  Bus Creator/1 -> Bus Selector2/1, Bus Selector1/1, Bus Selector/1, Bus Selector3/1
  Constant/1 -> Mux2/1, Mux1/2, Mux3/4, Mux4/3
  Bus Selector3/3 -> Gain 1/1  "<wy>"
  Gain 4/1 -> Mux2/2
  Gain 6/1 -> Mux2/3
  Bus Selector/2 -> Gain 6/1  "<wy>"
  Bus Selector/3 -> Gain 2/1  "<wz>"
  Dot Product 2/1 -> Mux6/4
  Dot Product 3/1 -> Mux6/3
  Dot Product 4/1 -> Mux6/2
  Dot Product 1/1 -> Mux6/1
  Demux/4 -> Dot Product 3/1, Dot Product 4/1, Dot Product 1/1, Dot Product 2/1
  Gain 7/1 -> d(Q)/dt/1
  Bus Selector3/1 -> Mux1/1  "<wx>"
  Bus Selector3/2 -> Mux1/3  "<wz>"
  Gain 1/1 -> Mux1/4
  Bus Selector1/3 -> Gain 3/1  "<wx>"
  Bus Selector1/2 -> Mux3/2  "<wy>"
  Bus Selector1/1 -> Mux3/1  "<wz>"
  Bus Selector2/1 -> Mux4/1  "<wy>"
  Bus Selector2/2 -> Gain 5/1  "<wz>"
  Bus Selector2/3 -> Mux4/4  "<wx>"

== system X31dynamics_03/12 ODEs/acceleration ==
  force : Inport
  mass : Inport  Port=2
  Mux : Mux  Inputs=2
  Mux1 : Mux  Inputs=3
  x : Fcn  Expr=u(1)/u(4)
  y : Fcn  Expr=u(2)/u(4)
  z : Fcn  Expr=u(3)/u(4)
  accel : Outport
  wires:
  force/1 -> Mux/1
  Mux/1 -> z/1, y/1, x/1
  Mux1/1 -> accel/1
  x/1 -> Mux1/1
  y/1 -> Mux1/2
  z/1 -> Mux1/3
  mass/1 -> Mux/2

== system X31dynamics_03/12 ODEs/position dot ==
  V earth : Inport
  Demux : Demux  Outputs=[3 3 3]
  Mux1 : Mux  Inputs=3
  Terminator1 : Terminator
  Terminator2 : Terminator
  Vx : Fcn  Expr=u(1)
  Vy : Fcn  Expr=u(2)
  Vz : Fcn  Expr=u(3)
  d(xyz)/dt : Outport
  wires:
  Mux1/1 -> d(xyz)/dt/1
  V earth/1 -> Demux/1
  Demux/3 -> Terminator1/1
  Demux/1 -> Terminator2/1
  Demux/2 -> Vz/1, Vx/1, Vy/1
  Vx/1 -> Mux1/1
  Vy/1 -> Mux1/2
  Vz/1 -> Mux1/3

== system X31dynamics_03/12 ODEs/rotational acceleration rotate dot ==
  note: 1 Mx My Mz
      | 4 Ix Iy Iz
      | 7p q r
  moment : Inport
  inertia : Inport  Port=2
  rotation : Inport  Port=3
  Demux1 : Demux  Outputs=[3 4]
  Mux : Mux  Inputs=3
  Mux1 : Mux  Inputs=3
  Terminator3 : Terminator
  p dot : Fcn  Expr=((u(5)-u(6))*u(8)*u(9) + u(1))/u(4)
  q dot : Fcn  Expr=((u(6)-u(4))*u(7)*u(9) + u(2)) / u(5)
  r dot : Fcn  Expr=((u(4)-u(5))*u(7)*u(8) + u(3)) / u(6)
  d(pqr)/dt : Outport
  wires:
  moment/1 -> Mux/1
  Mux/1 -> r dot/1, q dot/1, p dot/1
  Mux1/1 -> d(pqr)/dt/1
  p dot/1 -> Mux1/1
  q dot/1 -> Mux1/2
  r dot/1 -> Mux1/3
  inertia/1 -> Mux/2
  rotation/1 -> Demux1/1
  Demux1/1 -> Mux/3
  Demux1/2 -> Terminator3/1

== system X31dynamics_03/Vectors/1,0,0 ==
  Ixy : Constant  Value=0
  Ixz : Constant  Value=0
  Mux6 : Mux  Inputs=3
  m : Constant
  1,0,0 : Outport
  wires:
  Mux6/1 -> 1,0,0/1
  m/1 -> Mux6/1
  Ixy/1 -> Mux6/3
  Ixz/1 -> Mux6/2

== system X31dynamics_03/Vectors/1,0,1 ==
  Ixy : Constant  Value=0
  Ixz : Constant
  Mux6 : Mux  Inputs=3
  m : Constant  Value=0
  0,1,0 : Outport
  wires:
  Mux6/1 -> 0,1,0/1
  m/1 -> Mux6/1
  Ixy/1 -> Mux6/3
  Ixz/1 -> Mux6/2

== system X31dynamics_03/aerodynamic Forces/Drag coefficient (2.2.2) ==
  note: p   q   r
      | Q1-Q4
  note: Vinf alpha beta rho
  note: aero_coef Fb
      | CD0
  aero V value : Inport
  aero_coef Fb : Inport  Port=2
  stateR : Inport  Port=3
  Reverse : Inport  Port=4
  CD0 : Fcn  Expr=u(1)
  Terminator : Terminator
  Terminator1 : Terminator
  Terminator2 : Terminator
  ail prop F body : Display  Commented=on
  main wing F : Display  Commented=on
  stateR 2 : Display  Commented=on
  CD : Outport
  wires:
  CD0/1 -> CD/1
  stateR/1 -> Terminator/1
  Reverse/1 -> Terminator1/1
  aero_coef Fb/1 -> CD0/1
  aero V value/1 -> Terminator2/1

== system X31dynamics_03/aerodynamic Forces/Drag to body coordinate1 ==
  note: drag must pointing in opesite direction of airflow
  note: Vinf alpha beta rho
  Drag : Inport
  aero V : Inport  Port=2
  -x dir : Gain  Gain=-1
  Aero : Display
  Air to Body : Subsystem  AncestorBlock=QuaternionLib/Air to Body
      mask help: Earth to body by rotational matrix Mv
  Constant : Constant  Value=0
  Demux : Demux  Outputs=[1 1 1 1]
  Demux1 : Demux  Outputs=[1 1 1]
  Mux : Mux  Inputs=3
  Terminator : Terminator
  Terminator1 : Terminator
  xb : Outport
  yb : Outport  Port=2
  zb : Outport  Port=3
  wires:
  aero V/1 -> Demux/1
  Demux/2 -> Air to Body/1(alpha)
  Demux/3 -> Air to Body/2(beta)
  Demux/1 -> Terminator/1
  Demux/4 -> Terminator1/1
  Demux1/1 -> xb/1
  Demux1/2 -> yb/1
  Demux1/3 -> zb/1
  Mux/1 -> Air to Body/3(v)
  Constant/1 -> Mux/2, Mux/3
  Air to Body/1(Mv) -> Aero/1, Demux1/1
  Drag/1 -> -x dir/1
  -x dir/1 -> Mux/1

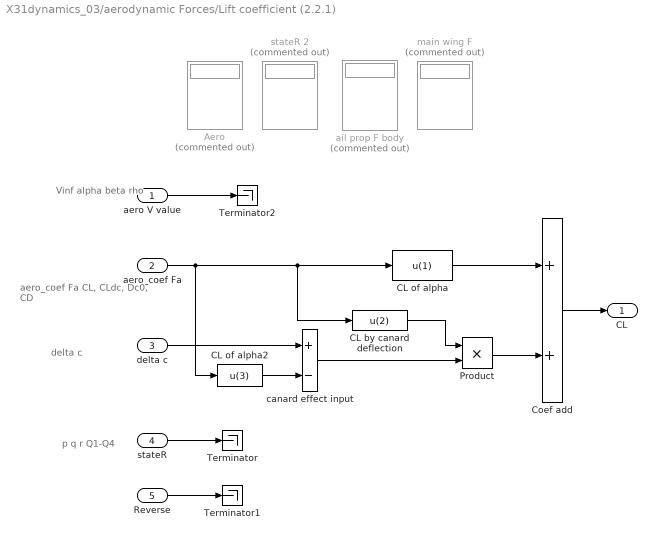
== system X31dynamics_03/aerodynamic Forces/Lift coefficient (2.2.1) ==
  note: p   q   r
      | Q1-Q4
  note: delta c
  note: Vinf alpha beta rho
  note: aero_coef Fa
      | CL, CLdc, Dc0, CD
  aero V value : Inport
  aero_coef Fa : Inport  Port=2
  delta c : Inport  Port=3
  stateR : Inport  Port=4
  Reverse : Inport  Port=5
  Aero : Display  Commented=on
  CL by canard deflection : Fcn  Expr=u(2)
  CL of alpha : Fcn  Expr=u(1)
  CL of alpha2 : Fcn  Expr=u(3)
  Coef add : Sum
  Product : Product
  Terminator : Terminator
  Terminator1 : Terminator
  Terminator2 : Terminator
  ail prop F body : Display  Commented=on
  canard effect input : Sum  Inputs=+-
  main wing F : Display  Commented=on
  stateR 2 : Display  Commented=on
  CL : Outport
  wires:
  Coef add/1 -> CL/1
  stateR/1 -> Terminator/1
  Reverse/1 -> Terminator1/1
  aero_coef Fa/1 -> CL of alpha/1, CL by canard deflection/1, CL of alpha2/1
  CL of alpha/1 -> Coef add/1
  aero V value/1 -> Terminator2/1
  CL by canard deflection/1 -> Product/1
  CL of alpha2/1 -> canard effect input/2
  delta c/1 -> canard effect input/1
  canard effect input/1 -> Product/2
  Product/1 -> Coef add/2

== system X31dynamics_03/aerodynamic Forces/Lift to body coordinate ==
  note: point up: -z
  Lift : Inport
  aero V : Inport  Port=2
  -cos( alpha ) : Fcn  Expr=-cos( u(2) )
  0 : Constant  Value=0
  Product : Product
  Product1 : Product
  sin( alpha ) : Fcn  Expr=sin( u(2) )
  xb : Outport
  yb : Outport  Port=2
  zb : Outport  Port=3
  wires:
  aero V/1 -> sin( alpha )/1, -cos( alpha )/1
  Product/1 -> xb/1
  Product1/1 -> zb/1
  -cos( alpha )/1 -> Product1/2
  sin( alpha )/1 -> Product/1
  0/1 -> yb/1
  Lift/1 -> Product1/1, Product/2

== system X31dynamics_03/aerodynamic Forces/Side force coefficient (2.2.3) ==
  note: 9 p   q   r
      | 12 Q1-Q4
  note: 1 Vinf alpha beta rho
  note: 5 CYb, CYda, CYdr
  note: 8 ail rud
  aero V value : Inport
  aero_coef Fc : Inport  Port=2
  ail & rud : Inport  Port=3
  stateR : Inport  Port=4
  Reverse : Inport  Port=5
  Aero : Display  Commented=on
  Coef add : Sum  Inputs=+++
  Mux : Mux
  Terminator1 : Terminator
  ail prop F body : Display  Commented=on
  ailron (2.2.3-2) : Fcn  Expr=u(6) * u(8)
  main wing F : Display  Commented=on
  rudder (2.2.3-3) : Fcn  Expr=u(7) * u(9)
  sideslip (2.2.3-1) : Fcn  Expr=u(5) * u(3)
  stateR 2 : Display  Commented=on
  CY : Outport
  wires:
  Coef add/1 -> CY/1
  stateR/1 -> Mux/4
  Reverse/1 -> Terminator1/1
  aero V value/1 -> Mux/1
  aero_coef Fc/1 -> Mux/2
  ail & rud/1 -> Mux/3
  Mux/1 -> rudder (2.2.3-3)/1, ailron (2.2.3-2)/1, sideslip (2.2.3-1)/1
  sideslip (2.2.3-1)/1 -> Coef add/1
  rudder (2.2.3-3)/1 -> Coef add/3
  ailron (2.2.3-2)/1 -> Coef add/2

== system X31dynamics_03/aerodynamic Forces/Sideforce to body coordinate2 ==
  Side F : Inport
  aero V : Inport  Port=2
  0 : Constant  Value=0
  Product : Product
  Product1 : Product
  cos( beta ) : Fcn  Expr=cos( u(3) )
  sin( beta ) : Fcn  Expr=-sin( u(3) )
  xb : Outport
  yb : Outport  Port=2
  zb : Outport  Port=3
  wires:
  aero V/1 -> sin( beta )/1, cos( beta )/1
  Product/1 -> xb/1
  Product1/1 -> yb/1
  cos( beta )/1 -> Product1/2
  Side F/1 -> Product1/1, Product/2
  sin( beta )/1 -> Product/1
  0/1 -> zb/1

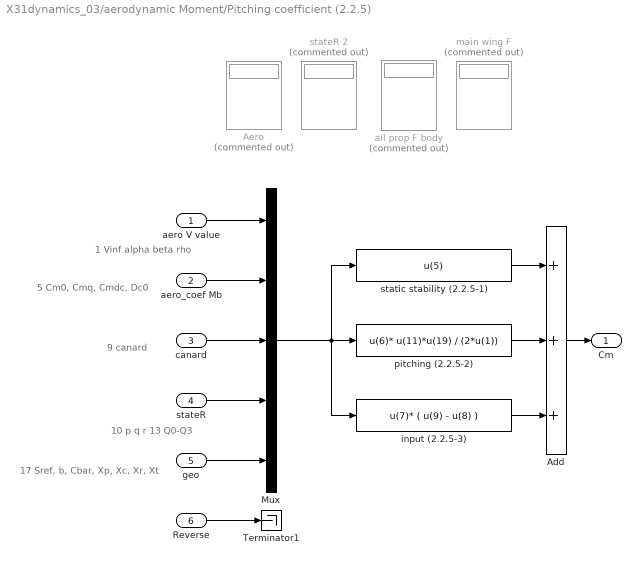
== system X31dynamics_03/aerodynamic Moment/Pitching coefficient (2.2.5) ==
  note: 9 canard
  note: 10 p   q   r
      | 13 Q0-Q3
  note: 1 Vinf alpha beta rho
  note: 17 Sref, b, Cbar, Xp, Xc, Xr, Xt
  note: 5 Cm0, Cmq, Cmdc, Dc0
  aero V value : Inport
  aero_coef Mb : Inport  Port=2
  canard : Inport  Port=3
  stateR : Inport  Port=4
  geo : Inport  Port=5
  Reverse : Inport  Port=6
  Add : Sum  Inputs=+++
  Aero : Display  Commented=on
  Mux : Mux  Inputs=5
  Terminator1 : Terminator
  ail prop F body : Display  Commented=on
  input (2.2.5-3) : Fcn  Expr=u(7)* ( u(9) - u(8) )
  main wing F : Display  Commented=on
  pitching (2.2.5-2) : Fcn  Expr=u(6)* u(11)*u(19) / (2*u(1))
  stateR 2 : Display  Commented=on
  static stability (2.2.5-1) : Fcn  Expr=u(5)
  Cm : Outport
  wires:
  Reverse/1 -> Terminator1/1
  aero_coef Mb/1 -> Mux/2
  Mux/1 -> static stability (2.2.5-1)/1, pitching (2.2.5-2)/1, input (2.2.5-3)/1
  aero V value/1 -> Mux/1
  canard/1 -> Mux/3
  stateR/1 -> Mux/4
  geo/1 -> Mux/5
  input (2.2.5-3)/1 -> Add/3
  pitching (2.2.5-2)/1 -> Add/2
  static stability (2.2.5-1)/1 -> Add/1
  Add/1 -> Cm/1

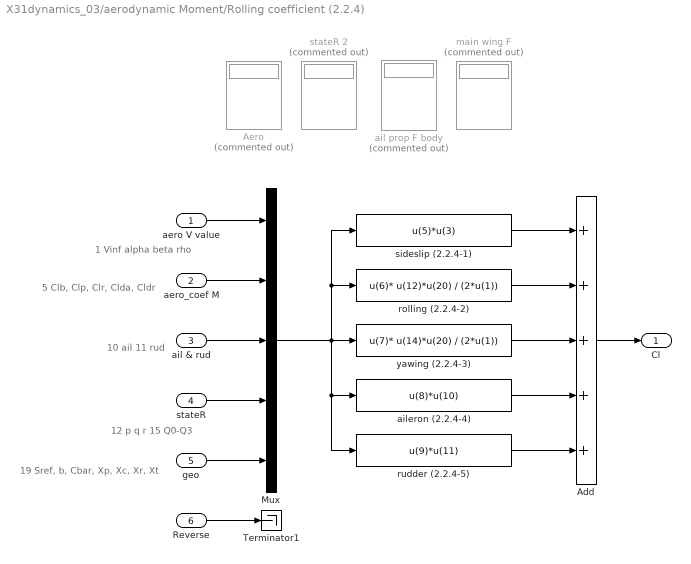
== system X31dynamics_03/aerodynamic Moment/Rolling coefficient (2.2.4) ==
  note: 10 ail
      | 11 rud
  note: 12 p   q   r
      | 15 Q0-Q3
  note: 1 Vinf alpha beta rho
  note: 5 Clb, Clp, Clr, Clda, Cldr
  note: 19 Sref, b, Cbar, Xp, Xc, Xr, Xt
  aero V value : Inport
  aero_coef M : Inport  Port=2
  ail & rud : Inport  Port=3
  stateR : Inport  Port=4
  geo : Inport  Port=5
  Reverse : Inport  Port=6
  Add : Sum  Inputs=+++++
  Aero : Display  Commented=on
  Mux : Mux  Inputs=5
  Terminator1 : Terminator
  ail prop F body : Display  Commented=on
  aileron (2.2.4-4) : Fcn  Expr=u(8)*u(10)
  main wing F : Display  Commented=on
  rolling (2.2.4-2) : Fcn  Expr=u(6)* u(12)*u(20) / (2*u(1))
  rudder (2.2.4-5) : Fcn  Expr=u(9)*u(11)
  sideslip (2.2.4-1) : Fcn  Expr=u(5)*u(3)
  stateR 2 : Display  Commented=on
  yawing (2.2.4-3) : Fcn  Expr=u(7)* u(14)*u(20) / (2*u(1))
  Cl : Outport
  wires:
  Reverse/1 -> Terminator1/1
  aero_coef M/1 -> Mux/2
  Mux/1 -> sideslip (2.2.4-1)/1, rolling (2.2.4-2)/1, yawing (2.2.4-3)/1, rudder (2.2.4-5)/1, aileron (2.2.4-4)/1
  aero V value/1 -> Mux/1
  ail & rud/1 -> Mux/3
  stateR/1 -> Mux/4
  geo/1 -> Mux/5
  rudder (2.2.4-5)/1 -> Add/5
  aileron (2.2.4-4)/1 -> Add/4
  yawing (2.2.4-3)/1 -> Add/3
  rolling (2.2.4-2)/1 -> Add/2
  sideslip (2.2.4-1)/1 -> Add/1
  Add/1 -> Cl/1

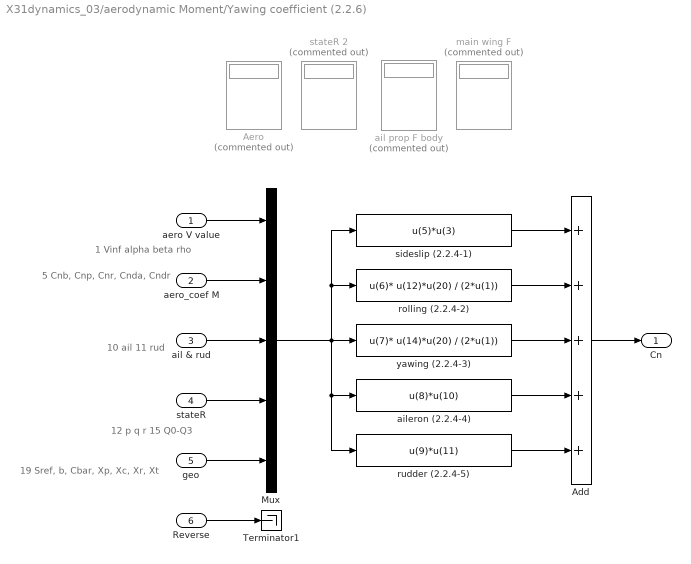
== system X31dynamics_03/aerodynamic Moment/Yawing coefficient (2.2.6) ==
  note: 10 ail
      | 11 rud
  note: 12 p   q   r
      | 15 Q0-Q3
  note: 1 Vinf alpha beta rho
  note: 19 Sref, b, Cbar, Xp, Xc, Xr, Xt
  note: 5 Cnb, Cnp, Cnr, Cnda, Cndr
  aero V value : Inport
  aero_coef M : Inport  Port=2
  ail & rud : Inport  Port=3
  stateR : Inport  Port=4
  geo : Inport  Port=5
  Reverse : Inport  Port=6
  Add : Sum  Inputs=+++++
  Aero : Display  Commented=on
  Mux : Mux  Inputs=5
  Terminator1 : Terminator
  ail prop F body : Display  Commented=on
  aileron (2.2.4-4) : Fcn  Expr=u(8)*u(10)
  main wing F : Display  Commented=on
  rolling (2.2.4-2) : Fcn  Expr=u(6)* u(12)*u(20) / (2*u(1))
  rudder (2.2.4-5) : Fcn  Expr=u(9)*u(11)
  sideslip (2.2.4-1) : Fcn  Expr=u(5)*u(3)
  stateR 2 : Display  Commented=on
  yawing (2.2.4-3) : Fcn  Expr=u(7)* u(14)*u(20) / (2*u(1))
  Cn : Outport
  wires:
  Reverse/1 -> Terminator1/1
  aero_coef M/1 -> Mux/2
  Mux/1 -> sideslip (2.2.4-1)/1, rolling (2.2.4-2)/1, yawing (2.2.4-3)/1, rudder (2.2.4-5)/1, aileron (2.2.4-4)/1
  aero V value/1 -> Mux/1
  ail & rud/1 -> Mux/3
  stateR/1 -> Mux/4
  geo/1 -> Mux/5
  rudder (2.2.4-5)/1 -> Add/5
  aileron (2.2.4-4)/1 -> Add/4
  yawing (2.2.4-3)/1 -> Add/3
  rolling (2.2.4-2)/1 -> Add/2
  sideslip (2.2.4-1)/1 -> Add/1
  Add/1 -> Cn/1

== system X31dynamics_03/aerodynamic Forces/Drag to body coordinate1/Air to Body ==
  alpha : Inport
  beta : Inport  Port=2
  v : Inport  Port=3
  0 : Constant  Value=0
  Body 3-2-1 to Q : QuaternionLib/Body 3-2-1 to Q
  Body to Earth : QuaternionLib/Body to Earth
  Gain : Gain  Gain=-1
  MATLAB Function : MATLAB Function  Commented=on  TreatAsAtomicUnit=on
  Mv : Outport
  wires:
  Body 3-2-1 to Q/1 -> Body to Earth/1
  Gain/1 -> Body 3-2-1 to Q/2
  v/1 -> Body to Earth/2
  0/1 -> Body 3-2-1 to Q/3
  beta/1 -> Body 3-2-1 to Q/1
  alpha/1 -> Gain/1
  Body to Earth/1 -> Mv/1

== matlab function X31dynamics_03/aerodynamic Forces/Drag to body coordinate1/Air to Body/MATLAB Function ==
  data: x1 input; Mv output; x2 input; x3 input; v input
function Mv = body321_tf(x1, x2, x3, v)
c1 = cos(x3);
s1 = sin(x3);
c2 = cos(x2);
s2 = sin(x2);
c3 = cos(x1);
s3 = sin(x1);
M = [   c1*c2 , c1*s2*s3 - c3*s1 , c1*s2*c3 + s3*s1 ;...
        s1*c2 , s1*s2*s3 + c3*c1 , s1*s2*c3 - s3*c1 ;...
        -s2   ,            c2*s3 ,            c2*c3     ];
Mv = (M * v) ;
end

== matlab function X31dynamics_03/coefficient/aerodynamic coefficient ==
  data: fa output; a input; fb output; X31_initP parameter
function [fa,fb] = aero_coef(a,X31_initP)
    fa = zeros(1,10);
    fb = zeros(1,10);
    a = 180 / pi * a;   % convert to degree for polynomials
    a_abs = abs(a);
    for i = 1:10
        fa(i) = X31_initP.fig2_2(i).a(6)*a_abs^6 + X31_initP.fig2_2(i).a(5)*a_abs^5 + X31_initP.fig2_2(i).a(4)*a_abs^4 +...
                X31_initP.fig2_2(i).a(3)*a_abs^3 + X31_initP.fig2_2(i).a(2)*a_abs^2 + X31_initP.fig2_2(i).a(1)*a_abs + X31_initP.fig2_2(i).a(7);

        fb(i) = X31_initP.fig2_2(i).b(6)*a_abs^6 + X31_initP.fig2_2(i).b(5)*a_abs^5 + X31_initP.fig2_2(i).b(4)*a_abs^4 +...
                X31_initP.fig2_2(i).b(3)*a_abs^3 + X31_initP.fig2_2(i).b(2)*a_abs^2 + X31_initP.fig2_2(i).b(1)*a_abs + X31_initP.fig2_2(i).b(7);
        % for odd functions
        if (a<0) 
            if (X31_initP.fig2_2(i).a(8) ==1)
                fa(i) = -fa(i) + 2*X31_initP.fig2_2(i).a(7);
            end
            if (X31_initP.fig2_2(i).b(8) ==1)
                fb(i) = -fb(i) + 2*X31_initP.fig2_2(i).b(7);
            end
        end
    end
end

%{
     Force
CL   (α) 2.2.1a Odd
CLdc (α) 2.2.2a Even
C0d  (α) 2.2.2/l0b Odd
CD   (α) 2.2.1b Even
CYp  (α) 2.2.3a Even
CYda (α) Set zero Not Shown Even
CYdr (α) 2.2.3b Even

     Moment
Clb  (α) 2.2.4a Even
Clp  (α) 2.2.5a Even
Clr  (α) 2.2.6a Odd
Clda (α) 2.2.7a Even
Cldr (α) 2.2.8a Even

Cm0  (α) 4.65% e unstable 2.2.9a Odd
Cmq  (α) 3 2.2.9b Even
Cmdc      2.2.10a Even
C0d  (α) 2.2.2/10b Odd

Cnb  (α) 2.2.4b Even
Cnp  (α) 2.2.5b Odd
Cnr  (α) 2.2.6b Even
Cnda (α) 2.2.7b Even
Cndr (α) 2.2.8b Even
%}
